simulink model "hough_accumulator"  (R2020a)
settings: Solver=FixedStepDiscrete  StartTime=0.0  StopTime=inf  RelTol=1e-3
InitFcn:
  | setup;
StopFcn:
  | stop;
values from neighbouring files (symbols this model uses):
  fs = 250e6    (= 250000000)    [setup.m]
  height = 480    [setup.m]
  inarray = Y    [setup.m]
  maxRho = ceil(sqrt((height/2)^2+(width/2)^2))    [setup.m]
  nRho = maxRho*2    [setup.m]
  nTheta = length(theta)    [setup.m]
  sobelThreshold = 30    [setup.m]
  width = 640    [setup.m]
libraries: library x9, hdlsllib x2, simulink x1, dspsrcs4 x1
settings Model: DataTypeOverride=Off  SimulationMode=rapid-accelerator  Creator=david  LastModifiedBy=david
settings OptimizationCC: BlockReduction=off  ConditionallyExecuteInputs=off  DefaultParameterBehavior=Inlined
settings DebuggingCC: AlgebraicLoopMsg=error  SingleTaskRateTransMsg=error
settings HardwareCC: ProdBitPerPointer=32  ProdBitPerSizeT=32  ProdBitPerPtrDiffT=32  ProdLargestAtomicFloat=None  ProdIntDivRoundTo=Undefined  ProdEndianess=Unspecified  ProdWordSize=32  ProdHWDeviceType=ASIC/FPGA->ASIC/FPGA  TargetBitPerPointer=64  TargetBitPerSizeT=64  TargetBitPerPtrDiffT=64  TargetLongLongMode=on  TargetIntDivRoundTo=Zero  TargetEndianess=LittleEndian  TargetWordSize=64  TargetHWDeviceType=Custom Processor->MATLAB Host Computer  ProdEqTarget=off

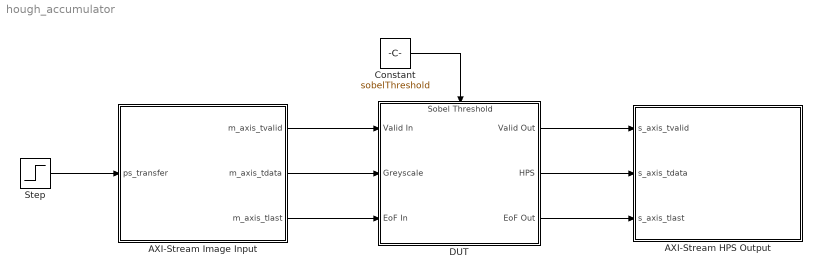
== system hough_accumulator ==
  AXI-Stream HPS Output : Subsystem  mask{height=nRho, width=nTheta, clk=1/fs, d=0}
      mask prompts: height "Image Height:"; width "Image Width:"; clk "Clock Rate:"; d "Frame Capture Number"
      mask DialogControl DescGroupVar Prompt: AXI-Stream Image Output
      mask DialogControl DescTextVar Prompt: Image output using the AXI-Stream interface. Simulates an AXI DMA write channel.
      mask DialogControl ParameterGroupVar Prompt: Main
  AXI-Stream Image Input : Subsystem  mask{image=inarray, clk=1/fs}
      mask prompts: image "Input Image:"; clk "Clock Rate:"
      mask init:
      | [height, width] = size(image);
      mask DialogControl DescGroupVar Prompt: AXI-Stream Image Input
      mask DialogControl DescTextVar Prompt: This block simulates an AXI-Stream image input for interfacing to a hardware accelerator or IP Core.
      mask DialogControl ParameterGroupVar Prompt: Main
  Constant : Constant  Value=sobelThreshold  OutDataTypeStr=uint32  SampleTime=-1
  DUT : Subsystem  TreatAsAtomicUnit=on
      settings: PortSchema="{\"entries\":[{\"content\":{\"sides\":[{\"content\":{\"connectorIds\":[\"In1\",\"In2\",\"In3\"]},\"type\":\"ConnectorPlacement.EquallySpacedRectSide\",\"uuid\":\"44ea3531-c301-49a5-8102-d6fa50cc6c19\"},{\"content\":{\"connectorIds\":[\"Out1\",\"Out2\",\"Out3\"],\"side\":\"RIGHT\"},\"type\":\"ConnectorPlacement.EquallySpacedRectSide\",\"uuid\":\"1d1c9d4f-057d-4585-815e-37c8ca7c240e\"},{\"content\":{\"connectorIds\":[\"In4\"],\"side\":\"TOP\"},\"type\":\"ConnectorPlacement.EquallySpacedRectSide\",\"uuid\":\"4593ddf2-7cbb-4da5-9369-2617dfadce47\"}]},\"type\":\"ConnectorPlacement.EquallySpacedConnector\",\"uuid\":\"b8449f0b-605c-4cae-8581-d877ef261dd9\"}],\"packageUris\":[\"http://schema.mathworks.com/mf0/Connector/19700101\"],\"version\":\"1.0\"}"
  Step : Step  Time=2/150e6  SampleTime=1/fs
  wires:
  DUT/3(EoF Out) -> AXI-Stream HPS Output/3(s_axis_tlast)
  DUT/1(Valid Out) -> AXI-Stream HPS Output/1(s_axis_tvalid)
  AXI-Stream Image Input/3(m_axis_tlast) -> DUT/3(EoF In)
  AXI-Stream Image Input/1(m_axis_tvalid) -> DUT/1(Valid In)
  AXI-Stream Image Input/2(m_axis_tdata) -> DUT/2(Greyscale)
  Step/1 -> AXI-Stream Image Input/1(ps_transfer)
  Constant/1 -> DUT/4(Sobel Threshold)
  DUT/2(HPS) -> AXI-Stream HPS Output/2(s_axis_tdata)

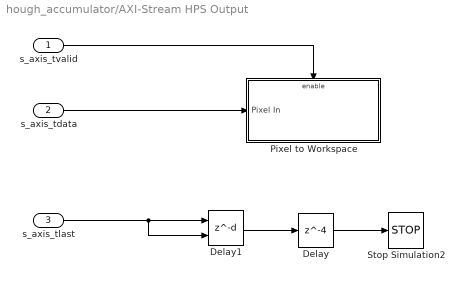
== system hough_accumulator/AXI-Stream HPS Output ==
  s_axis_tvalid : Inport
  s_axis_tdata : Inport  Port=2
  s_axis_tlast : Inport  Port=3
  Delay : Delay  DelayLength=4
  Delay1 : Delay  DelayLength=d  ShowEnablePort=on
      settings: InputPortMap=u0,e6
  Pixel to Workspace : Subsystem
  Stop Simulation2 : Stop
  wires:
  Delay/1 -> Stop Simulation2/1
  Delay1/1 -> Delay/1
  s_axis_tlast/1 -> Delay1/1, Delay1/2
  s_axis_tdata/1 -> Pixel to Workspace/1(Pixel In)
  s_axis_tvalid/1 -> Pixel to Workspace/Enable

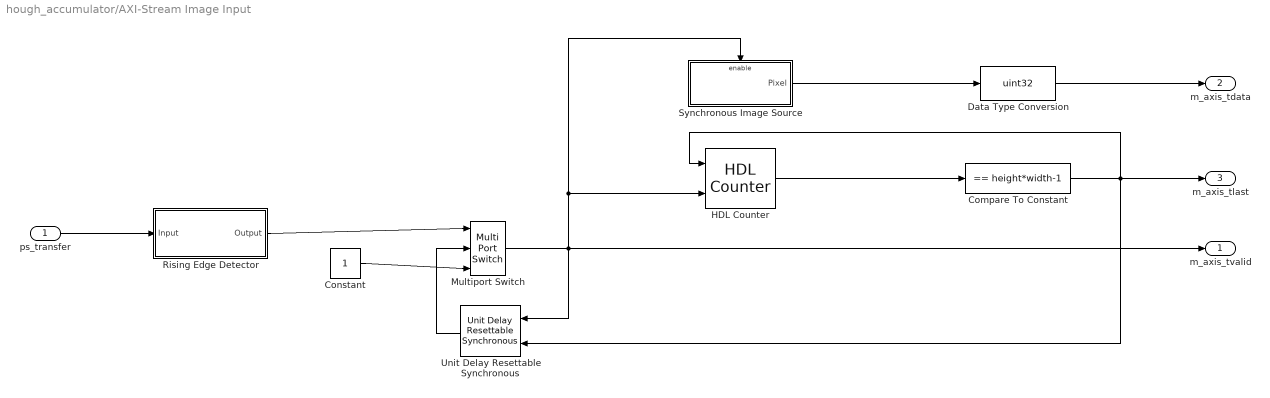
== system hough_accumulator/AXI-Stream Image Input ==
  ps_transfer : Inport
  Compare To Constant : simulink/Logic and Bit Operations/Compare To Constant  relop===  const=height*width-1  OutDataTypeStr=boolean
  Constant : Constant  OutDataTypeStr=boolean  SampleTime=-1
  Data Type Conversion : DataTypeConversion  OutDataTypeStr=uint32
  HDL Counter : hdlsllib/Sources/HDL Counter  CountType=Free running  CountInit=0  CountStep=1  CountMax=width*height-1  CountFromType=Initial value  CountFrom=0  CountResetPort=on  CountLoadPort=off  CountEnbPort=on  CountDirPort=off  CountDataType=Unsigned  CountWordLen=32  CountFracLen=0  CountSampTime=1
  Multiport Switch : MultiPortSwitch  DataPortOrder=Zero-based contiguous  Inputs=2  zeroidx=on
  Rising Edge Detector : Subsystem
  Synchronous Image Source : Subsystem
  Unit Delay Resettable Synchronous : hdlsllib/Discrete/Unit Delay Resettable Synchronous  InitialCondition=0.0  SampleTime=-1
      settings: SourceProductBaseCode=SL
  m_axis_tvalid : Outport
  m_axis_tdata : Outport  Port=2
  m_axis_tlast : Outport  Port=3
  wires:
  Constant/1 -> Multiport Switch/3
  Rising Edge Detector/1(Output) -> Multiport Switch/1
  Unit Delay Resettable Synchronous/1 -> Multiport Switch/2
  ps_transfer/1 -> Rising Edge Detector/1(Input)
  Data Type Conversion/1 -> m_axis_tdata/1
  Compare To Constant/1 -> m_axis_tlast/1, HDL Counter/1, Unit Delay Resettable Synchronous/2
  Multiport Switch/1 -> m_axis_tvalid/1, Synchronous Image Source/Enable, HDL Counter/2, Unit Delay Resettable Synchronous/1
  Synchronous Image Source/1(Pixel) -> Data Type Conversion/1
  HDL Counter/1 -> Compare To Constant/1

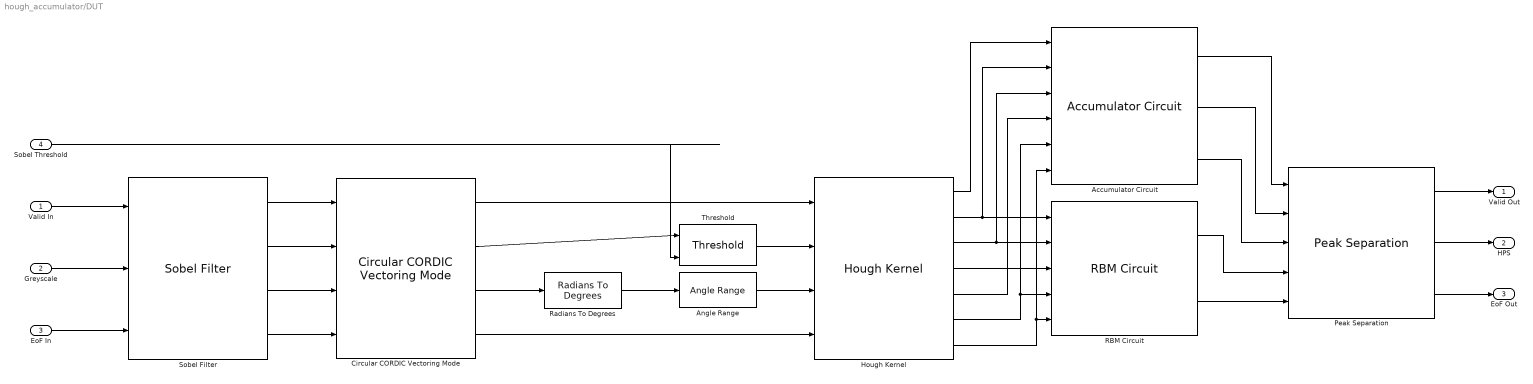
== system hough_accumulator/DUT ==
  Valid In : Inport
  Greyscale : Inport  Port=2
  EoF In : Inport  Port=3
  Sobel Threshold : Inport  Port=4
  Accumulator Circuit : library/Accumulator Circuit  height=height  width=width  rhoBits=ceil(log2(maxRho*2))  nTheta=nTheta  nRho=nRho
  Angle Range : library/Angle Range  SystemSampleTime=-1  Latency=0  AutoFrameSizeCalculation=off
  Circular CORDIC Vectoring Mode : library/Circular CORDIC Vectoring Mode  i=12  b=24  f=13
  Hough Kernel : library/Hough Kernel  rhoBits=ceil(log2(maxRho*2))  height=height  width=width  dTheta=1
  Peak Separation : library/Peak Separation  nRho=nRho  nTheta=nTheta
  RBM Circuit : library/RBM Circuit  height=height  width=width  nTheta=nTheta  rhoBits=ceil(log2(maxRho*2))  nRho=nRho
  Radians To Degrees : library/Radians To Degrees  f=0
  Sobel Filter : library/Sobel Filter  height=height  width=width
  Threshold : library/Threshold  b=11  f=0  s=0
  Valid Out : Outport  VectorParamsAs1DForOutWhenUnconnected=off
  HPS : Outport  Port=2  VectorParamsAs1DForOutWhenUnconnected=off
  EoF Out : Outport  Port=3  VectorParamsAs1DForOutWhenUnconnected=off
  wires:
  Valid In/1 -> Sobel Filter/1
  Greyscale/1 -> Sobel Filter/2
  EoF In/1 -> Sobel Filter/3
  Sobel Filter/1 -> Circular CORDIC Vectoring Mode/1
  Sobel Filter/2 -> Circular CORDIC Vectoring Mode/2
  Sobel Filter/3 -> Circular CORDIC Vectoring Mode/3
  Sobel Filter/4 -> Circular CORDIC Vectoring Mode/4
  Circular CORDIC Vectoring Mode/3 -> Radians To Degrees/1
  Radians To Degrees/1 -> Angle Range/1
  Circular CORDIC Vectoring Mode/2 -> Threshold/1
  Sobel Threshold/1 -> Threshold/2
  Angle Range/1 -> Hough Kernel/3
  Threshold/1 -> Hough Kernel/2
  Circular CORDIC Vectoring Mode/1 -> Hough Kernel/1
  Circular CORDIC Vectoring Mode/4 -> Hough Kernel/4
  Hough Kernel/1 -> Accumulator Circuit/1
  Hough Kernel/2 -> RBM Circuit/1, Accumulator Circuit/2
  Hough Kernel/3 -> RBM Circuit/2, Accumulator Circuit/3
  Hough Kernel/5 -> Accumulator Circuit/4
  Hough Kernel/6 -> RBM Circuit/4, Accumulator Circuit/5
  Hough Kernel/7 -> RBM Circuit/5, Accumulator Circuit/6
  Hough Kernel/4 -> RBM Circuit/3
  Accumulator Circuit/1 -> Peak Separation/1
  Accumulator Circuit/2 -> Peak Separation/2
  Accumulator Circuit/3 -> Peak Separation/3
  RBM Circuit/1 -> Peak Separation/4
  RBM Circuit/2 -> Peak Separation/5
  Peak Separation/1 -> Valid Out/1
  Peak Separation/2 -> HPS/1
  Peak Separation/3 -> EoF Out/1

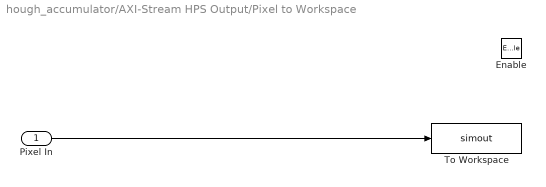
== system hough_accumulator/AXI-Stream HPS Output/Pixel to Workspace ==
  Pixel In : Inport
  Enable : EnablePort
  To Workspace : ToWorkspace  VariableName=simout  SampleTime=-1
      settings: MaxDataPoints=height*width  Save2DSignal=2-D array (concatenate along first dimension)
  wires:
  Pixel In/1 -> To Workspace/1

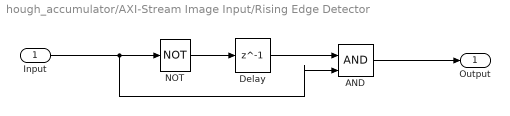
== system hough_accumulator/AXI-Stream Image Input/Rising Edge Detector ==
  Input : Inport
  AND : Logic  IconShape=distinctive  AllPortsSameDT=off  OutDataTypeStr=boolean
  Delay : Delay  DelayLength=1
  NOT : Logic  Operator=NOT  IconShape=distinctive  AllPortsSameDT=off  OutDataTypeStr=boolean
  Output : Outport  VectorParamsAs1DForOutWhenUnconnected=off
  wires:
  AND/1 -> Output/1
  Delay/1 -> AND/1
  Input/1 -> NOT/1, AND/2
  NOT/1 -> Delay/1

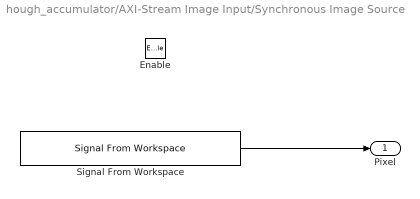
== system hough_accumulator/AXI-Stream Image Input/Synchronous Image Source ==
  Enable : EnablePort
  Signal From Workspace : dspsrcs4/Signal From Workspace  X=reshape(image', [height*width, 1])  Ts=clk  nsamps=1  OutputAfterFinalValue=Cyclic repetition  ignoreOrWarnInputAndFrameLengths=off  OutputFrames=off
  Pixel : Outport
  wires:
  Signal From Workspace/1 -> Pixel/1
